simulink library "lib_others"  (R2023a)
settings: Solver=VariableStepAuto  StartTime=0.0  StopTime=10.0  RelTol=1e-3
settings Model: Creator=FC_dev1  LastModifiedBy=FC_dev1

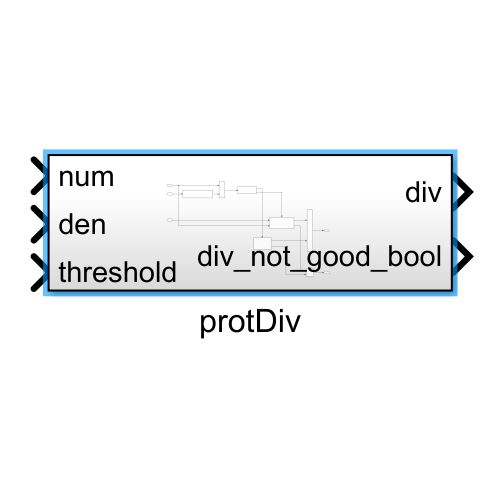
[thumbnail: Simulink's stored preview of the top-level diagram]
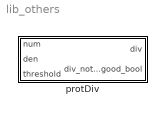
== system lib_others ==
  protDiv : Subsystem

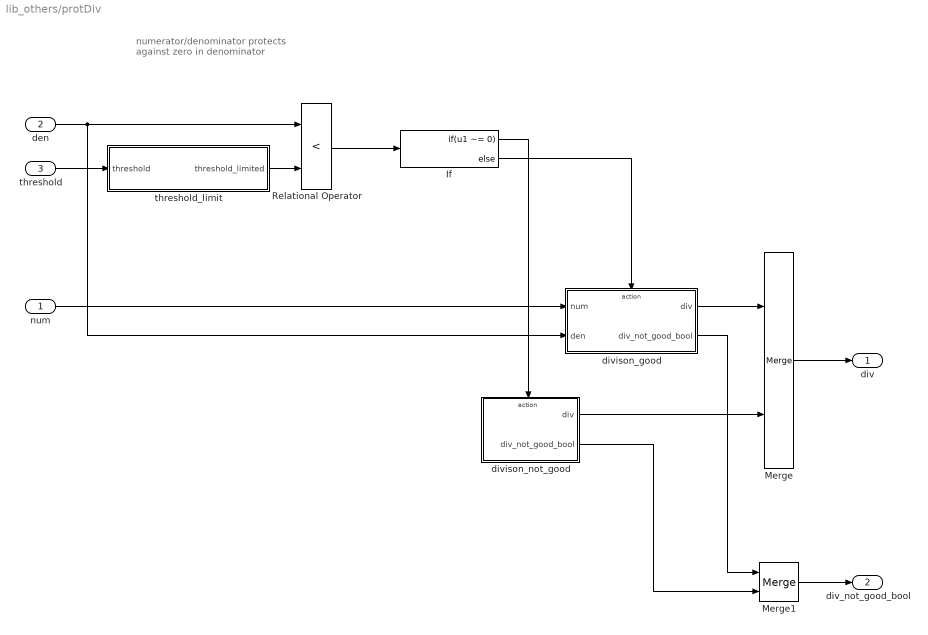
== system lib_others/protDiv ==
  note: numerator/denominator
      | protects against zero in denominator
  num : Inport  PortDimensions=1
  den : Inport  Port=2  PortDimensions=1
  threshold : Inport  Port=3  PortDimensions=1
  If : If  IfExpression=u1 ~= 0
  Merge : Merge
  Merge1 : Merge
  Relational Operator : RelationalOperator  Operator=<  OutDataTypeStr=boolean  RndMeth=Simplest  InputSameDT=off
  divison_good : Subsystem  TreatAsAtomicUnit=on
  divison_not_good : Subsystem  TreatAsAtomicUnit=on
  threshold_limit : Subsystem
  div : Outport  PortDimensions=1
  div_not_good_bool : Outport  Port=2  OutDataTypeStr=boolean  PortDimensions=1
  wires:
  num/1 -> divison_good/1(num)
  divison_good/1(div) -> Merge/1
  den/1 -> divison_good/2(den), Relational Operator/1
  threshold/1 -> threshold_limit/1(threshold)
  Relational Operator/1 -> If/1
  threshold_limit/1(threshold_limited) -> Relational Operator/2
  If/1 -> divison_not_good/Action
  If/2 -> divison_good/Action
  divison_not_good/1(div) -> Merge/2
  Merge/1 -> div/1
  divison_good/2(div_not_good_bool) -> Merge1/1
  divison_not_good/2(div_not_good_bool) -> Merge1/2
  Merge1/1 -> div_not_good_bool/1

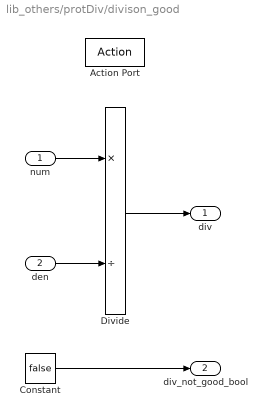
== system lib_others/protDiv/divison_good ==
  num : Inport
  den : Inport  Port=2
  Action Port : ActionPort  ActionPortLabel=else
  Constant : Constant  Value=false
  Divide : Product  Inputs=*/
  div : Outport
  div_not_good_bool : Outport  Port=2
  wires:
  Divide/1 -> div/1
  num/1 -> Divide/1
  den/1 -> Divide/2
  Constant/1 -> div_not_good_bool/1

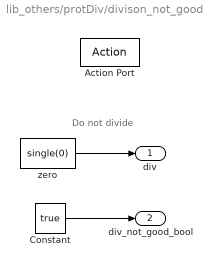
== system lib_others/protDiv/divison_not_good ==
  note: Do not divide
  Action Port : ActionPort  ActionPortLabel=if(u1 > 0)
  Constant : Constant  Value=true
  zero : Constant  Value=single(0)
  div : Outport
  div_not_good_bool : Outport  Port=2
  wires:
  zero/1 -> div/1
  Constant/1 -> div_not_good_bool/1

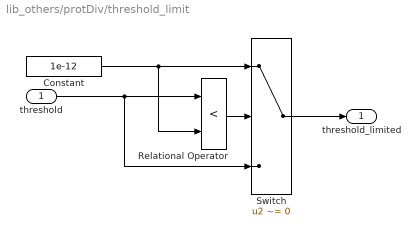
== system lib_others/protDiv/threshold_limit ==
  threshold : Inport
  Constant : Constant  Value=1e-12  OutDataTypeStr=Inherit: Inherit via back propagation
  Relational Operator : RelationalOperator  Operator=<  OutDataTypeStr=boolean  RndMeth=Simplest  InputSameDT=off
  Switch : Switch  Criteria=u2 ~= 0  SaturateOnIntegerOverflow=off  InputSameDT=off
  threshold_limited : Outport
  wires:
  threshold/1 -> Switch/3, Relational Operator/1
  Relational Operator/1 -> Switch/2
  Constant/1 -> Relational Operator/2, Switch/1
  Switch/1 -> threshold_limited/1
